simulink model "lab4"  (Simulink 7.1)
settings: Solver=ode45  StartTime=0.0  StopTime=100  RelTol=1e-3
settings Model: Creator=CARLOS BRUNO  LastModifiedBy=CARLOS BRUNO

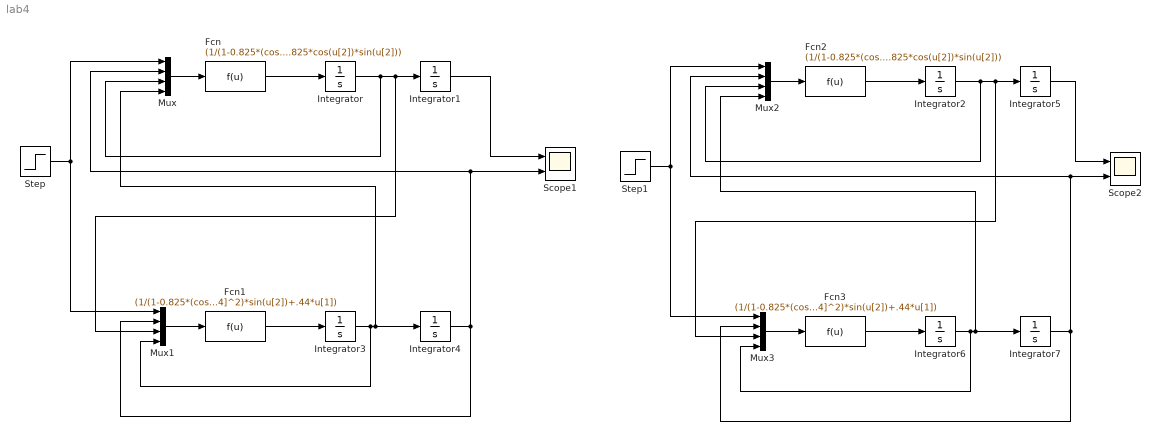
== system lab4 ==
  Fcn : Fcn  Expr=(1/(1-0.825*(cos(u[2])^2)))*(-.22*u[3] + .055*(u[4]^2)*sin(u[2]) + .825*cos(u[2])*sin(u[2]))
  Fcn1 : Fcn  Expr=(1/(1-0.825*(cos(u[2])^2)))*(14.71*sin(u[2])) - 1.5*cos(u[2])*(-.22*u[3] + .055*(u[4]^2)*sin(u[2])+.44*u[1])
  Fcn2 : Fcn  Expr=(1/(1-0.825*(cos(u[2])^2)))*(-.22*u[3] + .055*(u[4]^2)*sin(u[2]) + .825*cos(u[2])*sin(u[2]))
  Fcn3 : Fcn  Expr=(1/(1-0.825*(cos(u[2])^2)))*(14.71*sin(u[2])) - 1.5*cos(u[2])*(-.22*u[3] + .055*(u[4]^2)*sin(u[2])+.44*u[1])
  Integrator{,1..3,5..6} (6 alike) : Integrator
  Integrator4 : Integrator  InitialCondition=pi/3
  Integrator7 : Integrator  InitialCondition=pi/6
  Mux{,1..3} (4 alike) : Mux
  Scope1 : Scope  NumInputPorts=2
      settings: YMin=-5~-5  YMax=5~5
  Scope2 : Scope  NumInputPorts=2
      settings: YMin=-5~-5  YMax=5~5
  Step : Step  Time=0  After=0  SampleTime=0
  Step1 : Step  Time=0  After=0  SampleTime=0
  wires:
  Integrator/1 -> Mux/3, Integrator1/1, Mux1/3
  Integrator3/1 -> Integrator4/1, Mux/4, Mux1/4
  Fcn1/1 -> Integrator3/1
  Integrator4/1 -> Mux1/2, Mux/2, Scope1/2
  Step/1 -> Mux/1, Mux1/1
  Mux/1 -> Fcn/1
  Mux1/1 -> Fcn1/1
  Fcn/1 -> Integrator/1
  Integrator2/1 -> Mux2/3, Integrator5/1, Mux3/3
  Integrator6/1 -> Integrator7/1, Mux2/4, Mux3/4
  Fcn3/1 -> Integrator6/1
  Integrator7/1 -> Mux3/2, Mux2/2, Scope2/2
  Step1/1 -> Mux2/1, Mux3/1
  Mux2/1 -> Fcn2/1
  Mux3/1 -> Fcn3/1
  Fcn2/1 -> Integrator2/1
  Integrator1/1 -> Scope1/1
  Integrator5/1 -> Scope2/1
